simulink model "dynamicsSimulation"  (R2023a)
settings: Solver=VariableStepAuto  StartTime=0.0  StopTime=35  RelTol=1e-3
(part 1 of 2)
settings Model: Creator=eric  LastModifiedBy=eric

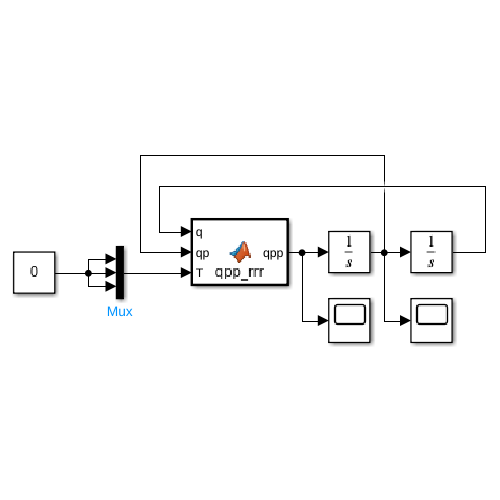
[thumbnail: Simulink's stored preview of the top-level diagram]
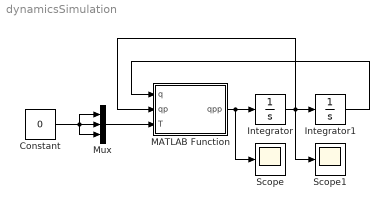
== system dynamicsSimulation ==
  Constant : Constant  Value=0
  Integrator : Integrator  InitialCondition=[0;0;0]
  Integrator1 : Integrator  InitialCondition=[0;pi/8;pi/4]
  MATLAB Function : MATLAB Function  TreatAsAtomicUnit=on
  Mux : Mux  Inputs=3
  Scope : Scope
  Scope1 : Scope
  wires:
  MATLAB Function/1(qpp) -> Scope/1, Integrator/1
  Integrator/1 -> Scope1/1, MATLAB Function/2(qp), Integrator1/1
  Integrator1/1 -> MATLAB Function/1(q)
  Constant/1 -> Mux/3, Mux/1, Mux/2
  Mux/1 -> MATLAB Function/3(T)
